simulink library "roller485lib"  (R2023a)
settings: Solver=VariableStepAuto  StartTime=0.0  StopTime=10.0  RelTol=1e-3
libraries: arduinolib x173, simulink x66
(part 3 of 6)

== system roller485lib/Basic I2C Write (using MATLAB Function)/basic angular velocity command [rpm] (using MATLAB Function) ==
  command [rpm] : Inport
  I2C Write (0x40) : arduinolib/I2C Write  I2CModule=0  Mode=Master  SlaveAddress=I2CAddress  SlaveByteOrder=BigEndian  Direction=Transmitter  RegisterAddressMode=on  RegisterAddress=0x40  SlaveDataType=uint8  DataLength=1  NoAck=off  RepeatedStart=off  OutputStatus=off  blockPlatform=ARDUINO
  MATLAB Function : MATLAB Function  TreatAsAtomicUnit=on
  x 100 : Gain  Gain=100
  wires:
  x 100/1 -> MATLAB Function/1(double_data)
  command [rpm]/1 -> x 100/1
  MATLAB Function/1(bytes) -> I2C Write (0x40)/1

== system roller485lib/Basic I2C Write (using MATLAB Function)/basic current command [A] (using MATLAB Function) ==
  command [A] : Inport
  A to mA : Gain  Gain=1000
  I2C Write (0xB0) : arduinolib/I2C Write  I2CModule=0  Mode=Master  SlaveAddress=I2CAddress  SlaveByteOrder=BigEndian  Direction=Transmitter  RegisterAddressMode=on  RegisterAddress=0xB0  SlaveDataType=uint8  DataLength=1  NoAck=off  RepeatedStart=off  OutputStatus=off  blockPlatform=ARDUINO
  MATLAB Function : MATLAB Function  TreatAsAtomicUnit=on
  x 100 : Gain  Gain=100
  wires:
  x 100/1 -> MATLAB Function/1(double_data)
  command [A]/1 -> A to mA/1
  MATLAB Function/1(bytes) -> I2C Write (0xB0)/1
  A to mA/1 -> x 100/1

== system roller485lib/Basic I2C Write (using MATLAB Function)/basic current command [mA] (using MATLAB Function) ==
  command [mA] : Inport
  I2C Write (0xB0) : arduinolib/I2C Write  I2CModule=0  Mode=Master  SlaveAddress=I2CAddress  SlaveByteOrder=BigEndian  Direction=Transmitter  RegisterAddressMode=on  RegisterAddress=0xB0  SlaveDataType=uint8  DataLength=1  NoAck=off  RepeatedStart=off  OutputStatus=off  blockPlatform=ARDUINO
  MATLAB Function : MATLAB Function  TreatAsAtomicUnit=on
  x 100 : Gain  Gain=100
  wires:
  MATLAB Function/1(bytes) -> I2C Write (0xB0)/1
  command [mA]/1 -> x 100/1
  x 100/1 -> MATLAB Function/1(double_data)

== system roller485lib/Basic I2C Write (using MATLAB Function)/basic relative angle command [deg] (using MATLAB Function) ==
  command [deg] : Inport
  Clock : Clock
  Compare To Constant : simulink/Logic and Bit Operations/Compare To Constant  relop===  const=0  OutDataTypeStr=boolean
  Enabled Subsystem (initialization angle) : Subsystem  TreatAsAtomicUnit=on
  I2C Write (0x80) : arduinolib/I2C Write  I2CModule=0  Mode=Master  SlaveAddress=I2CAddress  SlaveByteOrder=BigEndian  Direction=Transmitter  RegisterAddressMode=on  RegisterAddress=0x80  SlaveDataType=uint8  DataLength=1  NoAck=off  RepeatedStart=off  OutputStatus=off  blockPlatform=ARDUINO
  MATLAB Function : MATLAB Function  TreatAsAtomicUnit=on
  Sum : Sum  Inputs=++|
  x 100 : Gain  Gain=100
  wires:
  x 100/1 -> MATLAB Function/1(double_data)
  MATLAB Function/1(bytes) -> I2C Write (0x80)/1
  Compare To Constant/1 -> Enabled Subsystem (initialization angle)/Enable
  Clock/1 -> Compare To Constant/1
  command [deg]/1 -> Sum/2
  Enabled Subsystem (initialization angle)/1(initial angle) -> Sum/1
  Sum/1 -> x 100/1

== system roller485lib/Basic I2C Write (using MATLAB Function)/basic relative angle command [rad] (using MATLAB Function) ==
  command [rad] : Inport
  Clock : Clock
  Compare To Constant : simulink/Logic and Bit Operations/Compare To Constant  relop===  const=0  OutDataTypeStr=boolean
  Enabled Subsystem (initialization angle) : Subsystem  TreatAsAtomicUnit=on
  I2C Write (0x80) : arduinolib/I2C Write  I2CModule=0  Mode=Master  SlaveAddress=I2CAddress  SlaveByteOrder=BigEndian  Direction=Transmitter  RegisterAddressMode=on  RegisterAddress=0x80  SlaveDataType=uint8  DataLength=1  NoAck=off  RepeatedStart=off  OutputStatus=off  blockPlatform=ARDUINO
  MATLAB Function : MATLAB Function  TreatAsAtomicUnit=on
  Sum : Sum  Inputs=++|
  rad to deg : Gain  Gain=180/pi
  x 100 : Gain  Gain=100
  wires:
  Enabled Subsystem (initialization angle)/1(initial angle) -> Sum/1
  command [rad]/1 -> rad to deg/1
  Clock/1 -> Compare To Constant/1
  Compare To Constant/1 -> Enabled Subsystem (initialization angle)/Enable
  MATLAB Function/1(bytes) -> I2C Write (0x80)/1
  x 100/1 -> MATLAB Function/1(double_data)
  Sum/1 -> x 100/1
  rad to deg/1 -> Sum/2

== system roller485lib/Basic I2C Write (using MATLAB Function)/position PID (using MATLAB Function) ==
  " x 10^5 " : Gain  Gain=1e5
  D : Constant  Value=position_D
  I : Constant  Value=position_I
  I2C Write (0xA0) : arduinolib/I2C Write  I2CModule=0  Mode=Master  SlaveAddress=I2CAddress  SlaveByteOrder=BigEndian  Direction=Transmitter  RegisterAddressMode=on  RegisterAddress=0xA0  SlaveDataType=uint8  DataLength=1  NoAck=off  RepeatedStart=off  OutputStatus=off  blockPlatform=ARDUINO
  I2C Write (0xA4) : arduinolib/I2C Write  I2CModule=0  Mode=Master  SlaveAddress=I2CAddress  SlaveByteOrder=BigEndian  Direction=Transmitter  RegisterAddressMode=on  RegisterAddress=0xA4  SlaveDataType=uint8  DataLength=1  NoAck=off  RepeatedStart=off  OutputStatus=off  blockPlatform=ARDUINO
  I2C Write (0xA8) : arduinolib/I2C Write  I2CModule=0  Mode=Master  SlaveAddress=I2CAddress  SlaveByteOrder=BigEndian  Direction=Transmitter  RegisterAddressMode=on  RegisterAddress=0xA8  SlaveDataType=uint8  DataLength=1  NoAck=off  RepeatedStart=off  OutputStatus=off  blockPlatform=ARDUINO
  MATLAB Function (D) : MATLAB Function  TreatAsAtomicUnit=on
  MATLAB Function (I) : MATLAB Function  TreatAsAtomicUnit=on
  MATLAB Function (P) : MATLAB Function  TreatAsAtomicUnit=on
  P : Constant  Value=position_P
  x 10^5 : Gain  Gain=1e5
  x 10^7 : Gain  Gain=1e7
  wires:
  x 10^5/1 -> MATLAB Function (P)/1(double_data)
  MATLAB Function (P)/1(bytes) -> I2C Write (0xA0)/1
  P/1 -> x 10^5/1
  I/1 -> x 10^7/1
  MATLAB Function (I)/1(bytes) -> I2C Write (0xA4)/1
  x 10^7/1 -> MATLAB Function (I)/1(double_data)
  " x 10^5 "/1 -> MATLAB Function (D)/1(double_data)
  MATLAB Function (D)/1(bytes) -> I2C Write (0xA8)/1
  D/1 -> " x 10^5 "/1

== system roller485lib/Basic I2C Write (using MATLAB Function)/position PID (within set time) (using MATLAB Function) ==
  Clock : Clock
  Compare To Constant : simulink/Logic and Bit Operations/Compare To Constant  relop=<=  const=set_time  OutDataTypeStr=boolean
  D : Constant  Value=position_D
  Enabled Subsystem : Subsystem  TreatAsAtomicUnit=on
  I : Constant  Value=position_I
  P : Constant  Value=position_P
  wires:
  D/1 -> Enabled Subsystem/3(D)
  I/1 -> Enabled Subsystem/2(I)
  P/1 -> Enabled Subsystem/1(P)
  Compare To Constant/1 -> Enabled Subsystem/Enable
  Clock/1 -> Compare To Constant/1

== system roller485lib/Basic I2C Write (using MATLAB Function)/speed PID (using MATLAB Function) ==
  " x 10^5 " : Gain  Gain=1e5
  D : Constant  Value=speed_D
  I : Constant  Value=speed_I
  I2C Write (0x70) : arduinolib/I2C Write  I2CModule=0  Mode=Master  SlaveAddress=I2CAddress  SlaveByteOrder=BigEndian  Direction=Transmitter  RegisterAddressMode=on  RegisterAddress=0x70  SlaveDataType=uint8  DataLength=1  NoAck=off  RepeatedStart=off  OutputStatus=off  blockPlatform=ARDUINO
  I2C Write (0x74) : arduinolib/I2C Write  I2CModule=0  Mode=Master  SlaveAddress=I2CAddress  SlaveByteOrder=BigEndian  Direction=Transmitter  RegisterAddressMode=on  RegisterAddress=0x74  SlaveDataType=uint8  DataLength=1  NoAck=off  RepeatedStart=off  OutputStatus=off  blockPlatform=ARDUINO
  I2C Write (0x78) : arduinolib/I2C Write  I2CModule=0  Mode=Master  SlaveAddress=I2CAddress  SlaveByteOrder=BigEndian  Direction=Transmitter  RegisterAddressMode=on  RegisterAddress=0x78  SlaveDataType=uint8  DataLength=1  NoAck=off  RepeatedStart=off  OutputStatus=off  blockPlatform=ARDUINO
  MATLAB Function (D) : MATLAB Function  TreatAsAtomicUnit=on
  MATLAB Function (I) : MATLAB Function  TreatAsAtomicUnit=on
  MATLAB Function (P) : MATLAB Function  TreatAsAtomicUnit=on
  P : Constant  Value=speed_P
  x 10^5 : Gain  Gain=1e5
  x 10^7 : Gain  Gain=1e7
  wires:
  D/1 -> " x 10^5 "/1
  MATLAB Function (D)/1(bytes) -> I2C Write (0x78)/1
  " x 10^5 "/1 -> MATLAB Function (D)/1(double_data)
  x 10^7/1 -> MATLAB Function (I)/1(double_data)
  MATLAB Function (I)/1(bytes) -> I2C Write (0x74)/1
  I/1 -> x 10^7/1
  P/1 -> x 10^5/1
  MATLAB Function (P)/1(bytes) -> I2C Write (0x70)/1
  x 10^5/1 -> MATLAB Function (P)/1(double_data)

== system roller485lib/Basic I2C Write (using MATLAB Function)/speed PID (within set time) (using MATLAB Function) ==
  Clock : Clock
  Compare To Constant : simulink/Logic and Bit Operations/Compare To Constant  relop=<=  const=set_time  OutDataTypeStr=boolean
  D : Constant  Value=speed_D
  Enabled Subsystem : Subsystem  TreatAsAtomicUnit=on
  I : Constant  Value=speed_I
  P : Constant  Value=speed_P
  wires:
  Compare To Constant/1 -> Enabled Subsystem/Enable
  P/1 -> Enabled Subsystem/1(P)
  I/1 -> Enabled Subsystem/2(I)
  D/1 -> Enabled Subsystem/3(D)
  Clock/1 -> Compare To Constant/1

== system roller485lib/I2C Read/absolute angle detection [deg] ==
  Data Type Conversion : DataTypeConversion  OutDataTypeStr=double  SaturateOnIntegerOverflow=off  RndMeth=Floor
  I2C Read (0x90) : arduinolib/I2C Read  I2CModule=0  Mode=Master  SlaveAddress=I2CAddress  SlaveByteOrder=LittleEndian  Direction=Receiver  RegisterAddressMode=on  RegisterAddress=0x90  SlaveDataType=int32  DataLength=1  NoAck=off  RepeatedStart=off  OutputStatus=off  blockPlatform=ARDUINO  SampleTime=sample_time
  Reshape : Reshape
  x (1/100) : Gain  Gain=1/100
  deg : Outport
  wires:
  x (1/100)/1 -> Reshape/1
  I2C Read (0x90)/1 -> Data Type Conversion/1
  Data Type Conversion/1 -> x (1/100)/1
  Reshape/1 -> deg/1

== system roller485lib/I2C Read/absolute angle detection [rad] ==
  Data Type Conversion : DataTypeConversion  OutDataTypeStr=double  SaturateOnIntegerOverflow=off  RndMeth=Floor
  I2C Read (0x90) : arduinolib/I2C Read  I2CModule=0  Mode=Master  SlaveAddress=I2CAddress  SlaveByteOrder=LittleEndian  Direction=Receiver  RegisterAddressMode=on  RegisterAddress=0x90  SlaveDataType=int32  DataLength=1  NoAck=off  RepeatedStart=off  OutputStatus=off  blockPlatform=ARDUINO  SampleTime=sample_time
  Reshape : Reshape
  deg to rad : Gain  Gain=pi/180
  x (1/100) : Gain  Gain=1/100
  rad : Outport
  wires:
  x (1/100)/1 -> deg to rad/1
  deg to rad/1 -> Reshape/1
  Data Type Conversion/1 -> x (1/100)/1
  I2C Read (0x90)/1 -> Data Type Conversion/1
  Reshape/1 -> rad/1

== system roller485lib/I2C Read/angular velocity detection using LPF [rad//s] ==
  Data Type Conversion : DataTypeConversion  OutDataTypeStr=double  SaturateOnIntegerOverflow=off  RndMeth=Floor
  I2C Read (0x60) : arduinolib/I2C Read  I2CModule=0  Mode=Master  SlaveAddress=I2CAddress  SlaveByteOrder=LittleEndian  Direction=Receiver  RegisterAddressMode=on  RegisterAddress=0x60  SlaveDataType=int32  DataLength=1  NoAck=off  RepeatedStart=off  OutputStatus=off  blockPlatform=ARDUINO  SampleTime=sample_time
  Reshape : Reshape
  rpm to rad/s : Gain  Gain=2*pi/60
  x (1/100) : Gain  Gain=1/100
  rad/s : Outport
  wires:
  x (1/100)/1 -> rpm to rad/s/1
  rpm to rad/s/1 -> Reshape/1
  I2C Read (0x60)/1 -> Data Type Conversion/1
  Data Type Conversion/1 -> x (1/100)/1
  Reshape/1 -> rad/s/1

== system roller485lib/I2C Read/angular velocity detection using LPF [rpm] ==
  Data Type Conversion : DataTypeConversion  OutDataTypeStr=double  SaturateOnIntegerOverflow=off  RndMeth=Floor
  I2C Read (0x60) : arduinolib/I2C Read  I2CModule=0  Mode=Master  SlaveAddress=I2CAddress  SlaveByteOrder=LittleEndian  Direction=Receiver  RegisterAddressMode=on  RegisterAddress=0x60  SlaveDataType=int32  DataLength=1  NoAck=off  RepeatedStart=off  OutputStatus=off  blockPlatform=ARDUINO  SampleTime=sample_time
  Reshape : Reshape
  x (1/100) : Gain  Gain=1/100
  rpm : Outport
  wires:
  x (1/100)/1 -> Reshape/1
  Data Type Conversion/1 -> x (1/100)/1
  I2C Read (0x60)/1 -> Data Type Conversion/1
  Reshape/1 -> rpm/1

== system roller485lib/I2C Read/current detection [A] ==
  Data Type Conversion : DataTypeConversion  OutDataTypeStr=double  SaturateOnIntegerOverflow=off  RndMeth=Floor
  I2C Read (0xC0) : arduinolib/I2C Read  I2CModule=0  Mode=Master  SlaveAddress=I2CAddress  SlaveByteOrder=LittleEndian  Direction=Receiver  RegisterAddressMode=on  RegisterAddress=0xC0  SlaveDataType=int32  DataLength=1  NoAck=off  RepeatedStart=off  OutputStatus=off  blockPlatform=ARDUINO  SampleTime=sample_time
  Reshape : Reshape
  mA to A : Gain  Gain=1/1000
  x (1/100) : Gain  Gain=1/100
  A : Outport
  wires:
  x (1/100)/1 -> mA to A/1
  Data Type Conversion/1 -> x (1/100)/1
  mA to A/1 -> Reshape/1
  I2C Read (0xC0)/1 -> Data Type Conversion/1
  Reshape/1 -> A/1

== system roller485lib/I2C Read/current detection [mA] ==
  Data Type Conversion : DataTypeConversion  OutDataTypeStr=double  SaturateOnIntegerOverflow=off  RndMeth=Floor
  I2C Read (0xC0) : arduinolib/I2C Read  I2CModule=0  Mode=Master  SlaveAddress=I2CAddress  SlaveByteOrder=LittleEndian  Direction=Receiver  RegisterAddressMode=on  RegisterAddress=0xC0  SlaveDataType=int32  DataLength=1  NoAck=off  RepeatedStart=off  OutputStatus=off  blockPlatform=ARDUINO  SampleTime=sample_time
  Reshape : Reshape
  x (1/100) : Gain  Gain=1/100
  mA : Outport
  wires:
  Data Type Conversion/1 -> x (1/100)/1
  x (1/100)/1 -> Reshape/1
  I2C Read (0xC0)/1 -> Data Type Conversion/1
  Reshape/1 -> mA/1

== system roller485lib/I2C Read/relative angle detection [deg] ==
  Clock : Clock
  Compare To Constant : simulink/Logic and Bit Operations/Compare To Constant  relop=<=  const=set_time  OutDataTypeStr=boolean
  Data Type Conversion : DataTypeConversion  OutDataTypeStr=double  SaturateOnIntegerOverflow=off  RndMeth=Floor
  Enabled Subsystem (initialization of angle) : Subsystem  TreatAsAtomicUnit=on
  I2C Read (0x90) : arduinolib/I2C Read  I2CModule=0  Mode=Master  SlaveAddress=I2CAddress  SlaveByteOrder=LittleEndian  Direction=Receiver  RegisterAddressMode=on  RegisterAddress=0x90  SlaveDataType=int32  DataLength=1  NoAck=off  RepeatedStart=off  OutputStatus=off  blockPlatform=ARDUINO  SampleTime=sample_time
  Reshape : Reshape
  Sum : Sum  Inputs=-+|
  x (1/100) : Gain  Gain=1/100
  deg : Outport
  wires:
  Sum/1 -> x (1/100)/1
  Enabled Subsystem (initialization of angle)/1(phim(0)) -> Sum/1
  Data Type Conversion/1 -> Sum/2, Enabled Subsystem (initialization of angle)/1(phim)
  Clock/1 -> Compare To Constant/1
  x (1/100)/1 -> Reshape/1
  I2C Read (0x90)/1 -> Data Type Conversion/1
  Reshape/1 -> deg/1
  Compare To Constant/1 -> Enabled Subsystem (initialization of angle)/Enable

== system roller485lib/I2C Read/relative angle detection [rad] ==
  Clock : Clock
  Compare To Constant : simulink/Logic and Bit Operations/Compare To Constant  relop=<=  const=set_time  OutDataTypeStr=boolean
  Data Type Conversion : DataTypeConversion  OutDataTypeStr=double  SaturateOnIntegerOverflow=off  RndMeth=Floor
  Enabled Subsystem (initialization of angle) : Subsystem  TreatAsAtomicUnit=on
  I2C Read (0x90) : arduinolib/I2C Read  I2CModule=0  Mode=Master  SlaveAddress=I2CAddress  SlaveByteOrder=LittleEndian  Direction=Receiver  RegisterAddressMode=on  RegisterAddress=0x90  SlaveDataType=int32  DataLength=1  NoAck=off  RepeatedStart=off  OutputStatus=off  blockPlatform=ARDUINO  SampleTime=sample_time
  Reshape : Reshape
  Sum : Sum  Inputs=-+|
  deg to rad : Gain  Gain=pi/180
  x (1/100) : Gain  Gain=1/100
  rad : Outport
  wires:
  x (1/100)/1 -> deg to rad/1
  Clock/1 -> Compare To Constant/1
  Data Type Conversion/1 -> Enabled Subsystem (initialization of angle)/1(phim), Sum/2
  Enabled Subsystem (initialization of angle)/1(phim(0)) -> Sum/1
  Sum/1 -> x (1/100)/1
  deg to rad/1 -> Reshape/1
  I2C Read (0x90)/1 -> Data Type Conversion/1
  Reshape/1 -> rad/1
  Compare To Constant/1 -> Enabled Subsystem (initialization of angle)/Enable

== system roller485lib/I2C Read (using MATLAB Function)/absolute angle detection [deg] (using MATLAB Function) ==
  I2C Read (0x90) : arduinolib/I2C Read  I2CModule=0  Mode=Master  SlaveAddress=I2CAddress  SlaveByteOrder=BigEndian  Direction=Receiver  RegisterAddressMode=on  RegisterAddress=0x90  SlaveDataType=uint8  DataLength=4  NoAck=off  RepeatedStart=off  OutputStatus=off  blockPlatform=ARDUINO  SampleTime=sample_time
  MATLAB Function : MATLAB Function  TreatAsAtomicUnit=on
  x (1/100) : Gain  Gain=1/100
  deg : Outport
  wires:
  x (1/100)/1 -> deg/1
  MATLAB Function/1(double_data) -> x (1/100)/1
  I2C Read (0x90)/1 -> MATLAB Function/1(bytes)

== system roller485lib/I2C Read (using MATLAB Function)/absolute angle detection [rad] (using MATLAB Function) ==
  I2C Read (0x90) : arduinolib/I2C Read  I2CModule=0  Mode=Master  SlaveAddress=I2CAddress  SlaveByteOrder=BigEndian  Direction=Receiver  RegisterAddressMode=on  RegisterAddress=0x90  SlaveDataType=uint8  DataLength=4  NoAck=off  RepeatedStart=off  OutputStatus=off  blockPlatform=ARDUINO  SampleTime=sample_time
  MATLAB Function : MATLAB Function  TreatAsAtomicUnit=on
  deg to rad : Gain  Gain=pi/180
  x (1/100) : Gain  Gain=1/100
  rad : Outport
  wires:
  I2C Read (0x90)/1 -> MATLAB Function/1(bytes)
  MATLAB Function/1(double_data) -> x (1/100)/1
  x (1/100)/1 -> deg to rad/1
  deg to rad/1 -> rad/1

== system roller485lib/I2C Read (using MATLAB Function)/angular velocity detection using LPF [rad//s] (using MATLAB Function) ==
  I2C Read (0x60) : arduinolib/I2C Read  I2CModule=0  Mode=Master  SlaveAddress=I2CAddress  SlaveByteOrder=BigEndian  Direction=Receiver  RegisterAddressMode=on  RegisterAddress=0x60  SlaveDataType=uint8  DataLength=4  NoAck=off  RepeatedStart=off  OutputStatus=off  blockPlatform=ARDUINO  SampleTime=sample_time
  MATLAB Function2 : MATLAB Function  TreatAsAtomicUnit=on
  rpm to rad/s : Gain  Gain=2*pi/60
  x (1/100) : Gain  Gain=1/100
  rad/s : Outport
  wires:
  I2C Read (0x60)/1 -> MATLAB Function2/1(bytes)
  MATLAB Function2/1(double_data) -> x (1/100)/1
  x (1/100)/1 -> rpm to rad/s/1
  rpm to rad/s/1 -> rad/s/1

== system roller485lib/I2C Read (using MATLAB Function)/angular velocity detection using LPF [rpm] (using MATLAB Function) ==
  I2C Read (0x60) : arduinolib/I2C Read  I2CModule=0  Mode=Master  SlaveAddress=I2CAddress  SlaveByteOrder=BigEndian  Direction=Receiver  RegisterAddressMode=on  RegisterAddress=0x60  SlaveDataType=uint8  DataLength=4  NoAck=off  RepeatedStart=off  OutputStatus=off  blockPlatform=ARDUINO  SampleTime=sample_time
  MATLAB Function2 : MATLAB Function  TreatAsAtomicUnit=on
  x (1/100) : Gain  Gain=1/100
  rpm : Outport
  wires:
  x (1/100)/1 -> rpm/1
  MATLAB Function2/1(double_data) -> x (1/100)/1
  I2C Read (0x60)/1 -> MATLAB Function2/1(bytes)

== system roller485lib/I2C Read (using MATLAB Function)/current detection [A] (using MATLAB Function) ==
  I2C Read (0xC0) : arduinolib/I2C Read  I2CModule=0  Mode=Master  SlaveAddress=I2CAddress  SlaveByteOrder=BigEndian  Direction=Receiver  RegisterAddressMode=on  RegisterAddress=0xC0  SlaveDataType=uint8  DataLength=4  NoAck=off  RepeatedStart=off  OutputStatus=off  blockPlatform=ARDUINO  SampleTime=sample_time
  MATLAB Function : MATLAB Function  TreatAsAtomicUnit=on
  mA to A : Gain  Gain=1/1000
  x (1/100) : Gain  Gain=1/100
  A : Outport
  wires:
  x (1/100)/1 -> mA to A/1
  MATLAB Function/1(double_data) -> x (1/100)/1
  I2C Read (0xC0)/1 -> MATLAB Function/1(bytes)
  mA to A/1 -> A/1

== system roller485lib/I2C Read (using MATLAB Function)/current detection [mA] (using MATLAB Function) ==
  I2C Read (0xC0) : arduinolib/I2C Read  I2CModule=0  Mode=Master  SlaveAddress=I2CAddress  SlaveByteOrder=BigEndian  Direction=Receiver  RegisterAddressMode=on  RegisterAddress=0xC0  SlaveDataType=uint8  DataLength=4  NoAck=off  RepeatedStart=off  OutputStatus=off  blockPlatform=ARDUINO  SampleTime=sample_time
  MATLAB Function : MATLAB Function  TreatAsAtomicUnit=on
  x (1/100) : Gain  Gain=1/100
  mA : Outport
  wires:
  I2C Read (0xC0)/1 -> MATLAB Function/1(bytes)
  MATLAB Function/1(double_data) -> x (1/100)/1
  x (1/100)/1 -> mA/1

== system roller485lib/I2C Read (using MATLAB Function)/relative angle detection [deg] (using MATLAB Function) ==
  Clock : Clock
  Compare To Constant : simulink/Logic and Bit Operations/Compare To Constant  relop=<=  const=set_time  OutDataTypeStr=boolean
  Enabled Subsystem (initialization of angle) : Subsystem  TreatAsAtomicUnit=on
  I2C Read (0x90) : arduinolib/I2C Read  I2CModule=0  Mode=Master  SlaveAddress=I2CAddress  SlaveByteOrder=BigEndian  Direction=Receiver  RegisterAddressMode=on  RegisterAddress=0x90  SlaveDataType=uint8  DataLength=4  NoAck=off  RepeatedStart=off  OutputStatus=off  blockPlatform=ARDUINO  SampleTime=sample_time
  MATLAB Function : MATLAB Function  TreatAsAtomicUnit=on
  Sum : Sum  Inputs=-+|
  x (1/100) : Gain  Gain=1/100
  deg : Outport
  wires:
  Sum/1 -> x (1/100)/1
  Enabled Subsystem (initialization of angle)/1(phim(0)) -> Sum/1
  MATLAB Function/1(double_data) -> Sum/2, Enabled Subsystem (initialization of angle)/1(phim)
  Compare To Constant/1 -> Enabled Subsystem (initialization of angle)/Enable
  I2C Read (0x90)/1 -> MATLAB Function/1(bytes)
  x (1/100)/1 -> deg/1
  Clock/1 -> Compare To Constant/1

== system roller485lib/I2C Read (using MATLAB Function)/relative angle detection [rad] (using MATLAB Function) ==
  Clock : Clock
  Compare To Constant : simulink/Logic and Bit Operations/Compare To Constant  relop=<=  const=set_time  OutDataTypeStr=boolean
  Enabled Subsystem (initialization of angle) : Subsystem  TreatAsAtomicUnit=on
  I2C Read (0x90) : arduinolib/I2C Read  I2CModule=0  Mode=Master  SlaveAddress=I2CAddress  SlaveByteOrder=BigEndian  Direction=Receiver  RegisterAddressMode=on  RegisterAddress=0x90  SlaveDataType=uint8  DataLength=4  NoAck=off  RepeatedStart=off  OutputStatus=off  blockPlatform=ARDUINO  SampleTime=sample_time
  MATLAB Function : MATLAB Function  TreatAsAtomicUnit=on
  Sum : Sum  Inputs=-+|
  deg to rad : Gain  Gain=pi/180
  x (1/100) : Gain  Gain=1/100
  deg : Outport
  wires:
  x (1/100)/1 -> deg to rad/1
  I2C Read (0x90)/1 -> MATLAB Function/1(bytes)
  Compare To Constant/1 -> Enabled Subsystem (initialization of angle)/Enable
  MATLAB Function/1(double_data) -> Enabled Subsystem (initialization of angle)/1(phim), Sum/2
  Enabled Subsystem (initialization of angle)/1(phim(0)) -> Sum/1
  Sum/1 -> x (1/100)/1
  deg to rad/1 -> deg/1
  Clock/1 -> Compare To Constant/1

== system roller485lib/I2C Write/absolute angle command [deg] ==
  command [deg] : Inport
  Clock1 : Clock
  Clock2 : Clock
  Compare To Constant1 : simulink/Logic and Bit Operations/Compare To Constant  relop=<=  const=set_time1  OutDataTypeStr=boolean
  Compare To Constant2 : simulink/Logic and Bit Operations/Compare To Constant  relop=<=  const=set_time2  OutDataTypeStr=boolean
  D : Constant  Value=position_D
  Data Type Conversion : DataTypeConversion  OutDataTypeStr=uint32  SaturateOnIntegerOverflow=off  RndMeth=Floor
  Enabled Subsystem (PID setting) : Subsystem  TreatAsAtomicUnit=on
  Enabled Subsystem (mode setting) : Subsystem  TreatAsAtomicUnit=on
  I : Constant  Value=position_I
  I2C Write (0x80) : arduinolib/I2C Write  I2CModule=0  Mode=Master  SlaveAddress=I2CAddress  SlaveByteOrder=LittleEndian  Direction=Transmitter  RegisterAddressMode=on  RegisterAddress=0x80  SlaveDataType=uint8  DataLength=1  NoAck=off  RepeatedStart=off  OutputStatus=off  blockPlatform=ARDUINO
  P : Constant  Value=position_P
  position mode : Constant  Value=2
  x 100 : Gain  Gain=100
  wires:
  P/1 -> Enabled Subsystem (PID setting)/1(P)
  Clock1/1 -> Compare To Constant1/1
  position mode/1 -> Enabled Subsystem (mode setting)/1(mode)
  I/1 -> Enabled Subsystem (PID setting)/2(I)
  x 100/1 -> Data Type Conversion/1
  D/1 -> Enabled Subsystem (PID setting)/3(D)
  Compare To Constant2/1 -> Enabled Subsystem (PID setting)/Enable
  Compare To Constant1/1 -> Enabled Subsystem (mode setting)/Enable
  Clock2/1 -> Compare To Constant2/1
  Data Type Conversion/1 -> I2C Write (0x80)/1
  command [deg]/1 -> x 100/1

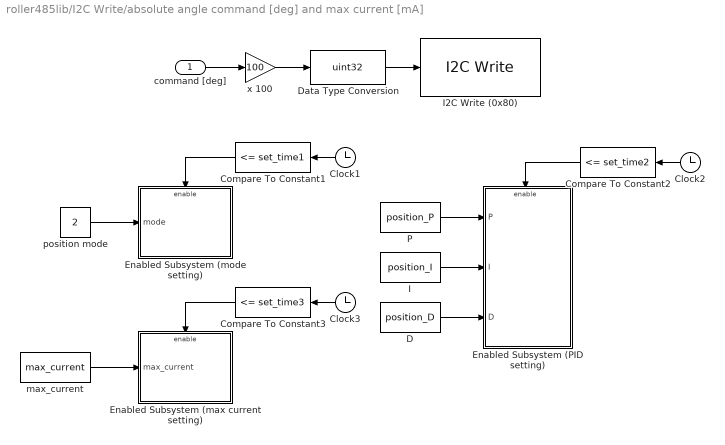
== system roller485lib/I2C Write/absolute angle command [deg] and max current [mA] ==
  command [deg] : Inport
  Clock1 : Clock
  Clock2 : Clock
  Clock3 : Clock
  Compare To Constant1 : simulink/Logic and Bit Operations/Compare To Constant  relop=<=  const=set_time1  OutDataTypeStr=boolean
  Compare To Constant2 : simulink/Logic and Bit Operations/Compare To Constant  relop=<=  const=set_time2  OutDataTypeStr=boolean
  Compare To Constant3 : simulink/Logic and Bit Operations/Compare To Constant  relop=<=  const=set_time3  OutDataTypeStr=boolean
  D : Constant  Value=position_D
  Data Type Conversion : DataTypeConversion  OutDataTypeStr=uint32  SaturateOnIntegerOverflow=off  RndMeth=Floor
  Enabled Subsystem (PID setting) : Subsystem  TreatAsAtomicUnit=on
  Enabled Subsystem (max current setting) : Subsystem  TreatAsAtomicUnit=on
  Enabled Subsystem (mode setting) : Subsystem  TreatAsAtomicUnit=on
  I : Constant  Value=position_I
  I2C Write (0x80) : arduinolib/I2C Write  I2CModule=0  Mode=Master  SlaveAddress=I2CAddress  SlaveByteOrder=LittleEndian  Direction=Transmitter  RegisterAddressMode=on  RegisterAddress=0x80  SlaveDataType=uint8  DataLength=1  NoAck=off  RepeatedStart=off  OutputStatus=off  blockPlatform=ARDUINO
  P : Constant  Value=position_P
  max_current : Constant  Value=max_current
  position mode : Constant  Value=2
  x 100 : Gain  Gain=100
  wires:
  P/1 -> Enabled Subsystem (PID setting)/1(P)
  Clock1/1 -> Compare To Constant1/1
  position mode/1 -> Enabled Subsystem (mode setting)/1(mode)
  I/1 -> Enabled Subsystem (PID setting)/2(I)
  Clock3/1 -> Compare To Constant3/1
  x 100/1 -> Data Type Conversion/1
  Compare To Constant3/1 -> Enabled Subsystem (max current setting)/Enable
  D/1 -> Enabled Subsystem (PID setting)/3(D)
  Compare To Constant2/1 -> Enabled Subsystem (PID setting)/Enable
  Compare To Constant1/1 -> Enabled Subsystem (mode setting)/Enable
  Clock2/1 -> Compare To Constant2/1
  max_current/1 -> Enabled Subsystem (max current setting)/1(max_current)
  Data Type Conversion/1 -> I2C Write (0x80)/1
  command [deg]/1 -> x 100/1

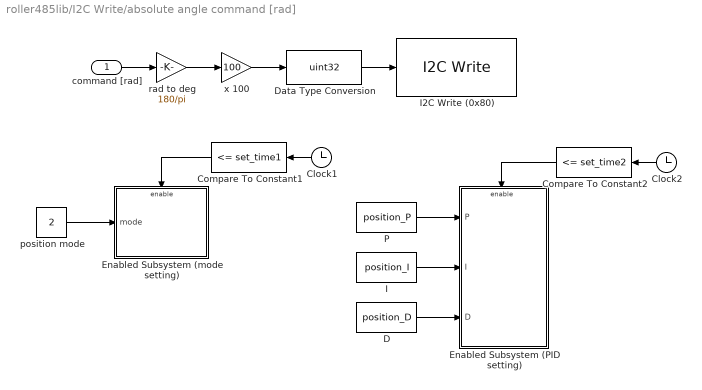
== system roller485lib/I2C Write/absolute angle command [rad] ==
  command [rad] : Inport
  Clock1 : Clock
  Clock2 : Clock
  Compare To Constant1 : simulink/Logic and Bit Operations/Compare To Constant  relop=<=  const=set_time1  OutDataTypeStr=boolean
  Compare To Constant2 : simulink/Logic and Bit Operations/Compare To Constant  relop=<=  const=set_time2  OutDataTypeStr=boolean
  D : Constant  Value=position_D
  Data Type Conversion : DataTypeConversion  OutDataTypeStr=uint32  SaturateOnIntegerOverflow=off  RndMeth=Floor
  Enabled Subsystem (PID setting) : Subsystem  TreatAsAtomicUnit=on
  Enabled Subsystem (mode setting) : Subsystem  TreatAsAtomicUnit=on
  I : Constant  Value=position_I
  I2C Write (0x80) : arduinolib/I2C Write  I2CModule=0  Mode=Master  SlaveAddress=I2CAddress  SlaveByteOrder=LittleEndian  Direction=Transmitter  RegisterAddressMode=on  RegisterAddress=0x80  SlaveDataType=uint8  DataLength=1  NoAck=off  RepeatedStart=off  OutputStatus=off  blockPlatform=ARDUINO
  P : Constant  Value=position_P
  position mode : Constant  Value=2
  rad to deg : Gain  Gain=180/pi
  x 100 : Gain  Gain=100
  wires:
  P/1 -> Enabled Subsystem (PID setting)/1(P)
  Clock1/1 -> Compare To Constant1/1
  position mode/1 -> Enabled Subsystem (mode setting)/1(mode)
  I/1 -> Enabled Subsystem (PID setting)/2(I)
  x 100/1 -> Data Type Conversion/1
  command [rad]/1 -> rad to deg/1
  D/1 -> Enabled Subsystem (PID setting)/3(D)
  Compare To Constant2/1 -> Enabled Subsystem (PID setting)/Enable
  Compare To Constant1/1 -> Enabled Subsystem (mode setting)/Enable
  Clock2/1 -> Compare To Constant2/1
  Data Type Conversion/1 -> I2C Write (0x80)/1
  rad to deg/1 -> x 100/1

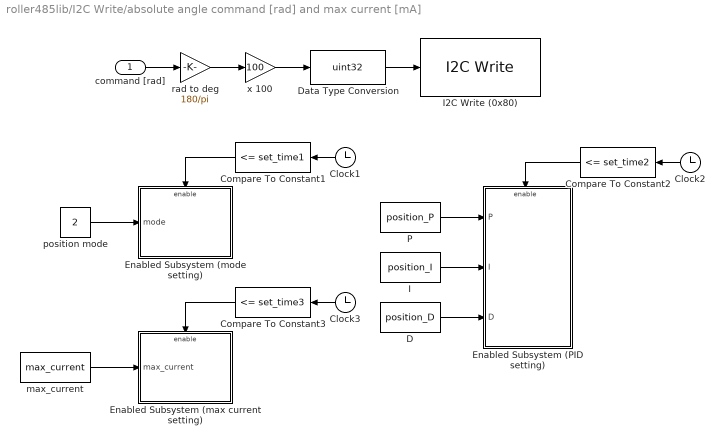
== system roller485lib/I2C Write/absolute angle command [rad] and max current [mA] ==
  command [rad] : Inport
  Clock1 : Clock
  Clock2 : Clock
  Clock3 : Clock
  Compare To Constant1 : simulink/Logic and Bit Operations/Compare To Constant  relop=<=  const=set_time1  OutDataTypeStr=boolean
  Compare To Constant2 : simulink/Logic and Bit Operations/Compare To Constant  relop=<=  const=set_time2  OutDataTypeStr=boolean
  Compare To Constant3 : simulink/Logic and Bit Operations/Compare To Constant  relop=<=  const=set_time3  OutDataTypeStr=boolean
  D : Constant  Value=position_D
  Data Type Conversion : DataTypeConversion  OutDataTypeStr=uint32  SaturateOnIntegerOverflow=off  RndMeth=Floor
  Enabled Subsystem (PID setting) : Subsystem  TreatAsAtomicUnit=on
  Enabled Subsystem (max current setting) : Subsystem  TreatAsAtomicUnit=on
  Enabled Subsystem (mode setting) : Subsystem  TreatAsAtomicUnit=on
  I : Constant  Value=position_I
  I2C Write (0x80) : arduinolib/I2C Write  I2CModule=0  Mode=Master  SlaveAddress=I2CAddress  SlaveByteOrder=LittleEndian  Direction=Transmitter  RegisterAddressMode=on  RegisterAddress=0x80  SlaveDataType=uint8  DataLength=1  NoAck=off  RepeatedStart=off  OutputStatus=off  blockPlatform=ARDUINO
  P : Constant  Value=position_P
  max_current : Constant  Value=max_current
  position mode : Constant  Value=2
  rad to deg : Gain  Gain=180/pi
  x 100 : Gain  Gain=100
  wires:
  command [rad]/1 -> rad to deg/1
  rad to deg/1 -> x 100/1
  Data Type Conversion/1 -> I2C Write (0x80)/1
  x 100/1 -> Data Type Conversion/1
  P/1 -> Enabled Subsystem (PID setting)/1(P)
  Clock1/1 -> Compare To Constant1/1
  Compare To Constant2/1 -> Enabled Subsystem (PID setting)/Enable
  I/1 -> Enabled Subsystem (PID setting)/2(I)
  D/1 -> Enabled Subsystem (PID setting)/3(D)
  Compare To Constant3/1 -> Enabled Subsystem (max current setting)/Enable
  Clock3/1 -> Compare To Constant3/1
  position mode/1 -> Enabled Subsystem (mode setting)/1(mode)
  max_current/1 -> Enabled Subsystem (max current setting)/1(max_current)
  Compare To Constant1/1 -> Enabled Subsystem (mode setting)/Enable
  Clock2/1 -> Compare To Constant2/1

== system roller485lib/I2C Write/angular velocity command [rad//s] ==
  command [rad/s] : Inport
  Clock1 : Clock
  Clock2 : Clock
  Compare To Constant1 : simulink/Logic and Bit Operations/Compare To Constant  relop=<=  const=set_time1  OutDataTypeStr=boolean
  Compare To Constant2 : simulink/Logic and Bit Operations/Compare To Constant  relop=<=  const=set_time2  OutDataTypeStr=boolean
  D : Constant  Value=speed_D
  Data Type Conversion : DataTypeConversion  OutDataTypeStr=uint32  SaturateOnIntegerOverflow=off  RndMeth=Floor
  Enabled Subsystem (PID setting) : Subsystem  TreatAsAtomicUnit=on
  Enabled Subsystem (mode setting) : Subsystem  TreatAsAtomicUnit=on
  I : Constant  Value=speed_I
  I2C Write (0x40) : arduinolib/I2C Write  I2CModule=0  Mode=Master  SlaveAddress=I2CAddress  SlaveByteOrder=LittleEndian  Direction=Transmitter  RegisterAddressMode=on  RegisterAddress=0x40  SlaveDataType=uint8  DataLength=1  NoAck=off  RepeatedStart=off  OutputStatus=off  blockPlatform=ARDUINO
  P : Constant  Value=speed_P
  rad/s to rpm : Gain  Gain=60/(2*pi)
  speed mode : Constant
  x 100 : Gain  Gain=100
  wires:
  command [rad/s]/1 -> rad/s to rpm/1
  rad/s to rpm/1 -> x 100/1
  Data Type Conversion/1 -> I2C Write (0x40)/1
  I/1 -> Enabled Subsystem (PID setting)/2(I)
  P/1 -> Enabled Subsystem (PID setting)/1(P)
  speed mode/1 -> Enabled Subsystem (mode setting)/1(mode)
  D/1 -> Enabled Subsystem (PID setting)/3(D)
  x 100/1 -> Data Type Conversion/1
  Compare To Constant1/1 -> Enabled Subsystem (mode setting)/Enable
  Clock2/1 -> Compare To Constant2/1
  Clock1/1 -> Compare To Constant1/1
  Compare To Constant2/1 -> Enabled Subsystem (PID setting)/Enable

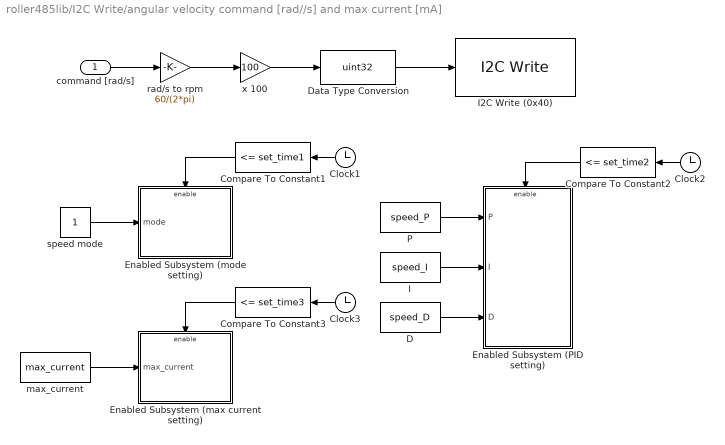
== system roller485lib/I2C Write/angular velocity command [rad//s] and max current [mA] ==
  command [rad/s] : Inport
  Clock1 : Clock
  Clock2 : Clock
  Clock3 : Clock
  Compare To Constant1 : simulink/Logic and Bit Operations/Compare To Constant  relop=<=  const=set_time1  OutDataTypeStr=boolean
  Compare To Constant2 : simulink/Logic and Bit Operations/Compare To Constant  relop=<=  const=set_time2  OutDataTypeStr=boolean
  Compare To Constant3 : simulink/Logic and Bit Operations/Compare To Constant  relop=<=  const=set_time3  OutDataTypeStr=boolean
  D : Constant  Value=speed_D
  Data Type Conversion : DataTypeConversion  OutDataTypeStr=uint32  SaturateOnIntegerOverflow=off  RndMeth=Floor
  Enabled Subsystem (PID setting) : Subsystem  TreatAsAtomicUnit=on
  Enabled Subsystem (max current setting) : Subsystem  TreatAsAtomicUnit=on
  Enabled Subsystem (mode setting) : Subsystem  TreatAsAtomicUnit=on
  I : Constant  Value=speed_I
  I2C Write (0x40) : arduinolib/I2C Write  I2CModule=0  Mode=Master  SlaveAddress=I2CAddress  SlaveByteOrder=LittleEndian  Direction=Transmitter  RegisterAddressMode=on  RegisterAddress=0x40  SlaveDataType=uint8  DataLength=1  NoAck=off  RepeatedStart=off  OutputStatus=off  blockPlatform=ARDUINO
  P : Constant  Value=speed_P
  max_current : Constant  Value=max_current
  rad/s to rpm : Gain  Gain=60/(2*pi)
  speed mode : Constant
  x 100 : Gain  Gain=100
  wires:
  command [rad/s]/1 -> rad/s to rpm/1
  rad/s to rpm/1 -> x 100/1
  Data Type Conversion/1 -> I2C Write (0x40)/1
  x 100/1 -> Data Type Conversion/1
  Clock2/1 -> Compare To Constant2/1
  Clock1/1 -> Compare To Constant1/1
  Clock3/1 -> Compare To Constant3/1
  Compare To Constant2/1 -> Enabled Subsystem (PID setting)/Enable
  D/1 -> Enabled Subsystem (PID setting)/3(D)
  I/1 -> Enabled Subsystem (PID setting)/2(I)
  P/1 -> Enabled Subsystem (PID setting)/1(P)
  max_current/1 -> Enabled Subsystem (max current setting)/1(max_current)
  speed mode/1 -> Enabled Subsystem (mode setting)/1(mode)
  Compare To Constant1/1 -> Enabled Subsystem (mode setting)/Enable
  Compare To Constant3/1 -> Enabled Subsystem (max current setting)/Enable

== system roller485lib/I2C Write/angular velocity command [rpm] ==
  command [rpm] : Inport
  Clock1 : Clock
  Clock2 : Clock
  Compare To Constant1 : simulink/Logic and Bit Operations/Compare To Constant  relop=<=  const=set_time1  OutDataTypeStr=boolean
  Compare To Constant2 : simulink/Logic and Bit Operations/Compare To Constant  relop=<=  const=set_time2  OutDataTypeStr=boolean
  D : Constant  Value=speed_D
  Data Type Conversion : DataTypeConversion  OutDataTypeStr=uint32  SaturateOnIntegerOverflow=off  RndMeth=Floor
  Enabled Subsystem (PID setting) : Subsystem  TreatAsAtomicUnit=on
  Enabled Subsystem (mode setting) : Subsystem  TreatAsAtomicUnit=on
  I : Constant  Value=speed_I
  I2C Write (0x40) : arduinolib/I2C Write  I2CModule=0  Mode=Master  SlaveAddress=I2CAddress  SlaveByteOrder=LittleEndian  Direction=Transmitter  RegisterAddressMode=on  RegisterAddress=0x40  SlaveDataType=uint8  DataLength=1  NoAck=off  RepeatedStart=off  OutputStatus=off  blockPlatform=ARDUINO
  P : Constant  Value=speed_P
  speed mode : Constant
  x 100 : Gain  Gain=100
  wires:
  Compare To Constant2/1 -> Enabled Subsystem (PID setting)/Enable
  Clock1/1 -> Compare To Constant1/1
  Clock2/1 -> Compare To Constant2/1
  Compare To Constant1/1 -> Enabled Subsystem (mode setting)/Enable
  x 100/1 -> Data Type Conversion/1
  D/1 -> Enabled Subsystem (PID setting)/3(D)
  speed mode/1 -> Enabled Subsystem (mode setting)/1(mode)
  P/1 -> Enabled Subsystem (PID setting)/1(P)
  I/1 -> Enabled Subsystem (PID setting)/2(I)
  Data Type Conversion/1 -> I2C Write (0x40)/1
  command [rpm]/1 -> x 100/1

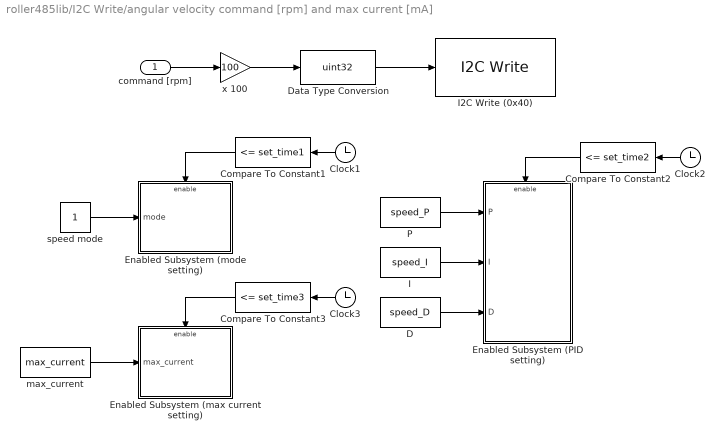
== system roller485lib/I2C Write/angular velocity command [rpm] and max current [mA] ==
  command [rpm] : Inport
  Clock1 : Clock
  Clock2 : Clock
  Clock3 : Clock
  Compare To Constant1 : simulink/Logic and Bit Operations/Compare To Constant  relop=<=  const=set_time1  OutDataTypeStr=boolean
  Compare To Constant2 : simulink/Logic and Bit Operations/Compare To Constant  relop=<=  const=set_time2  OutDataTypeStr=boolean
  Compare To Constant3 : simulink/Logic and Bit Operations/Compare To Constant  relop=<=  const=set_time3  OutDataTypeStr=boolean
  D : Constant  Value=speed_D
  Data Type Conversion : DataTypeConversion  OutDataTypeStr=uint32  SaturateOnIntegerOverflow=off  RndMeth=Floor
  Enabled Subsystem (PID setting) : Subsystem  TreatAsAtomicUnit=on
  Enabled Subsystem (max current setting) : Subsystem  TreatAsAtomicUnit=on
  Enabled Subsystem (mode setting) : Subsystem  TreatAsAtomicUnit=on
  I : Constant  Value=speed_I
  I2C Write (0x40) : arduinolib/I2C Write  I2CModule=0  Mode=Master  SlaveAddress=I2CAddress  SlaveByteOrder=LittleEndian  Direction=Transmitter  RegisterAddressMode=on  RegisterAddress=0x40  SlaveDataType=uint8  DataLength=1  NoAck=off  RepeatedStart=off  OutputStatus=off  blockPlatform=ARDUINO
  P : Constant  Value=speed_P
  max_current : Constant  Value=max_current
  speed mode : Constant
  x 100 : Gain  Gain=100
  wires:
  x 100/1 -> Data Type Conversion/1
  D/1 -> Enabled Subsystem (PID setting)/3(D)
  speed mode/1 -> Enabled Subsystem (mode setting)/1(mode)
  P/1 -> Enabled Subsystem (PID setting)/1(P)
  I/1 -> Enabled Subsystem (PID setting)/2(I)
  Data Type Conversion/1 -> I2C Write (0x40)/1
  command [rpm]/1 -> x 100/1
  max_current/1 -> Enabled Subsystem (max current setting)/1(max_current)
  Compare To Constant3/1 -> Enabled Subsystem (max current setting)/Enable
  Compare To Constant1/1 -> Enabled Subsystem (mode setting)/Enable
  Clock2/1 -> Compare To Constant2/1
  Clock1/1 -> Compare To Constant1/1
  Compare To Constant2/1 -> Enabled Subsystem (PID setting)/Enable
  Clock3/1 -> Compare To Constant3/1

== system roller485lib/I2C Write/current command [A] ==
  command [A] : Inport
  A to mA : Gain  Gain=1000
  "Clock " : Clock
  Compare To Constant : simulink/Logic and Bit Operations/Compare To Constant  relop=<=  const=set_time  OutDataTypeStr=boolean
  Data Type Conversion : DataTypeConversion  OutDataTypeStr=uint32  SaturateOnIntegerOverflow=off  RndMeth=Floor
  Enabled Subsystem (mode setting) : Subsystem  TreatAsAtomicUnit=on
  I2C Write (0xB0) : arduinolib/I2C Write  I2CModule=0  Mode=Master  SlaveAddress=I2CAddress  SlaveByteOrder=LittleEndian  Direction=Transmitter  RegisterAddressMode=on  RegisterAddress=0xB0  SlaveDataType=uint8  DataLength=1  NoAck=off  RepeatedStart=off  OutputStatus=off  blockPlatform=ARDUINO
  current mode : Constant  Value=3
  x 100 : Gain  Gain=100
  wires:
  x 100/1 -> Data Type Conversion/1
  command [A]/1 -> A to mA/1
  Data Type Conversion/1 -> I2C Write (0xB0)/1
  "Clock "/1 -> Compare To Constant/1
  Compare To Constant/1 -> Enabled Subsystem (mode setting)/Enable
  current mode/1 -> Enabled Subsystem (mode setting)/1(mode)
  A to mA/1 -> x 100/1

== system roller485lib/I2C Write/current command [mA] ==
  command [mA] : Inport
  "Clock " : Clock
  Compare To Constant : simulink/Logic and Bit Operations/Compare To Constant  relop=<=  const=set_time  OutDataTypeStr=boolean
  Data Type Conversion : DataTypeConversion  OutDataTypeStr=uint32  SaturateOnIntegerOverflow=off  RndMeth=Floor
  Enabled Subsystem (mode setting) : Subsystem  TreatAsAtomicUnit=on
  I2C Write (0xB0) : arduinolib/I2C Write  I2CModule=0  Mode=Master  SlaveAddress=I2CAddress  SlaveByteOrder=LittleEndian  Direction=Transmitter  RegisterAddressMode=on  RegisterAddress=0xB0  SlaveDataType=uint8  DataLength=1  NoAck=off  RepeatedStart=off  OutputStatus=off  blockPlatform=ARDUINO
  current mode : Constant  Value=3
  x 100 : Gain  Gain=100
  wires:
  current mode/1 -> Enabled Subsystem (mode setting)/1(mode)
  Compare To Constant/1 -> Enabled Subsystem (mode setting)/Enable
  "Clock "/1 -> Compare To Constant/1
  Data Type Conversion/1 -> I2C Write (0xB0)/1
  command [mA]/1 -> x 100/1
  x 100/1 -> Data Type Conversion/1

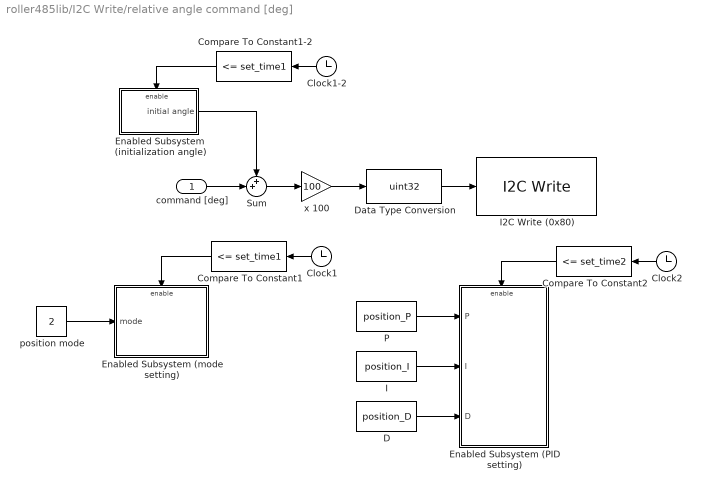
== system roller485lib/I2C Write/relative angle command [deg] ==
  command [deg] : Inport
  Clock1 : Clock
  Clock1-2 : Clock
  Clock2 : Clock
  Compare To Constant1 : simulink/Logic and Bit Operations/Compare To Constant  relop=<=  const=set_time1  OutDataTypeStr=boolean
  Compare To Constant1-2 : simulink/Logic and Bit Operations/Compare To Constant  relop=<=  const=set_time1  OutDataTypeStr=boolean
  Compare To Constant2 : simulink/Logic and Bit Operations/Compare To Constant  relop=<=  const=set_time2  OutDataTypeStr=boolean
  D : Constant  Value=position_D
  Data Type Conversion : DataTypeConversion  OutDataTypeStr=uint32  SaturateOnIntegerOverflow=off  RndMeth=Floor
  Enabled Subsystem (PID setting) : Subsystem  TreatAsAtomicUnit=on
  Enabled Subsystem (initialization angle) : Subsystem  TreatAsAtomicUnit=on
  Enabled Subsystem (mode setting) : Subsystem  TreatAsAtomicUnit=on
  I : Constant  Value=position_I
  I2C Write (0x80) : arduinolib/I2C Write  I2CModule=0  Mode=Master  SlaveAddress=I2CAddress  SlaveByteOrder=LittleEndian  Direction=Transmitter  RegisterAddressMode=on  RegisterAddress=0x80  SlaveDataType=uint8  DataLength=1  NoAck=off  RepeatedStart=off  OutputStatus=off  blockPlatform=ARDUINO
  P : Constant  Value=position_P
  Sum : Sum  Inputs=++|
  position mode : Constant  Value=2
  x 100 : Gain  Gain=100
  wires:
  Compare To Constant1-2/1 -> Enabled Subsystem (initialization angle)/Enable
  command [deg]/1 -> Sum/2
  Enabled Subsystem (initialization angle)/1(initial angle) -> Sum/1
  x 100/1 -> Data Type Conversion/1
  Sum/1 -> x 100/1
  Compare To Constant2/1 -> Enabled Subsystem (PID setting)/Enable
  position mode/1 -> Enabled Subsystem (mode setting)/1(mode)
  P/1 -> Enabled Subsystem (PID setting)/1(P)
  Clock1/1 -> Compare To Constant1/1
  Compare To Constant1/1 -> Enabled Subsystem (mode setting)/Enable
  Data Type Conversion/1 -> I2C Write (0x80)/1
  D/1 -> Enabled Subsystem (PID setting)/3(D)
  I/1 -> Enabled Subsystem (PID setting)/2(I)
  Clock2/1 -> Compare To Constant2/1
  Clock1-2/1 -> Compare To Constant1-2/1

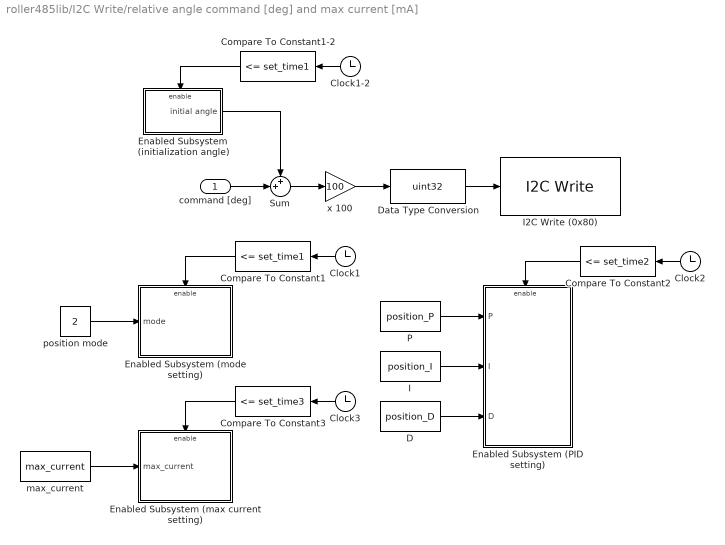
== system roller485lib/I2C Write/relative angle command [deg] and max current [mA] ==
  command [deg] : Inport
  Clock1 : Clock
  Clock1-2 : Clock
  Clock2 : Clock
  Clock3 : Clock
  Compare To Constant1 : simulink/Logic and Bit Operations/Compare To Constant  relop=<=  const=set_time1  OutDataTypeStr=boolean
  Compare To Constant1-2 : simulink/Logic and Bit Operations/Compare To Constant  relop=<=  const=set_time1  OutDataTypeStr=boolean
  Compare To Constant2 : simulink/Logic and Bit Operations/Compare To Constant  relop=<=  const=set_time2  OutDataTypeStr=boolean
  Compare To Constant3 : simulink/Logic and Bit Operations/Compare To Constant  relop=<=  const=set_time3  OutDataTypeStr=boolean
  D : Constant  Value=position_D
  Data Type Conversion : DataTypeConversion  OutDataTypeStr=uint32  SaturateOnIntegerOverflow=off  RndMeth=Floor
  Enabled Subsystem (PID setting) : Subsystem  TreatAsAtomicUnit=on
  Enabled Subsystem (initialization angle) : Subsystem  TreatAsAtomicUnit=on
  Enabled Subsystem (max current setting) : Subsystem  TreatAsAtomicUnit=on
  Enabled Subsystem (mode setting) : Subsystem  TreatAsAtomicUnit=on
  I : Constant  Value=position_I
  I2C Write (0x80) : arduinolib/I2C Write  I2CModule=0  Mode=Master  SlaveAddress=I2CAddress  SlaveByteOrder=LittleEndian  Direction=Transmitter  RegisterAddressMode=on  RegisterAddress=0x80  SlaveDataType=uint8  DataLength=1  NoAck=off  RepeatedStart=off  OutputStatus=off  blockPlatform=ARDUINO
  P : Constant  Value=position_P
  Sum : Sum  Inputs=++|
  max_current : Constant  Value=max_current
  position mode : Constant  Value=2
  x 100 : Gain  Gain=100
  wires:
  Compare To Constant1-2/1 -> Enabled Subsystem (initialization angle)/Enable
  command [deg]/1 -> Sum/2
  Enabled Subsystem (initialization angle)/1(initial angle) -> Sum/1
  x 100/1 -> Data Type Conversion/1
  Sum/1 -> x 100/1
  max_current/1 -> Enabled Subsystem (max current setting)/1(max_current)
  Compare To Constant2/1 -> Enabled Subsystem (PID setting)/Enable
  Compare To Constant3/1 -> Enabled Subsystem (max current setting)/Enable
  position mode/1 -> Enabled Subsystem (mode setting)/1(mode)
  P/1 -> Enabled Subsystem (PID setting)/1(P)
  Clock1/1 -> Compare To Constant1/1
  Compare To Constant1/1 -> Enabled Subsystem (mode setting)/Enable
  Data Type Conversion/1 -> I2C Write (0x80)/1
  D/1 -> Enabled Subsystem (PID setting)/3(D)
  I/1 -> Enabled Subsystem (PID setting)/2(I)
  Clock3/1 -> Compare To Constant3/1
  Clock2/1 -> Compare To Constant2/1
  Clock1-2/1 -> Compare To Constant1-2/1

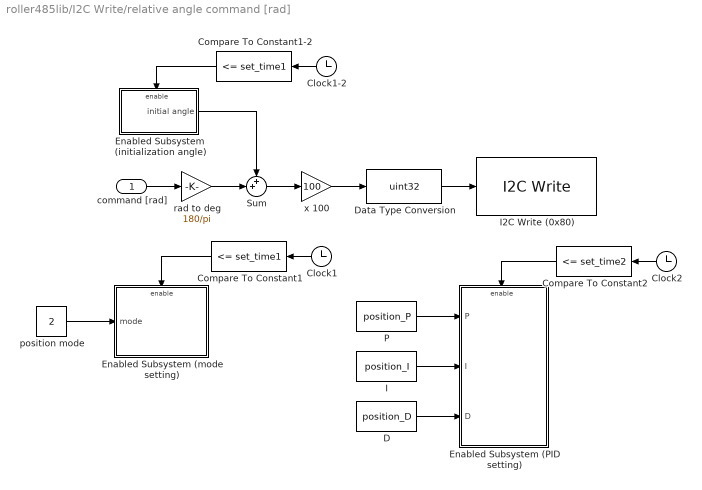
== system roller485lib/I2C Write/relative angle command [rad] ==
  command [rad] : Inport
  Clock1 : Clock
  Clock1-2 : Clock
  Clock2 : Clock
  Compare To Constant1 : simulink/Logic and Bit Operations/Compare To Constant  relop=<=  const=set_time1  OutDataTypeStr=boolean
  Compare To Constant1-2 : simulink/Logic and Bit Operations/Compare To Constant  relop=<=  const=set_time1  OutDataTypeStr=boolean
  Compare To Constant2 : simulink/Logic and Bit Operations/Compare To Constant  relop=<=  const=set_time2  OutDataTypeStr=boolean
  D : Constant  Value=position_D
  Data Type Conversion : DataTypeConversion  OutDataTypeStr=uint32  SaturateOnIntegerOverflow=off  RndMeth=Floor
  Enabled Subsystem (PID setting) : Subsystem  TreatAsAtomicUnit=on
  Enabled Subsystem (initialization angle) : Subsystem  TreatAsAtomicUnit=on
  Enabled Subsystem (mode setting) : Subsystem  TreatAsAtomicUnit=on
  I : Constant  Value=position_I
  I2C Write (0x80) : arduinolib/I2C Write  I2CModule=0  Mode=Master  SlaveAddress=I2CAddress  SlaveByteOrder=LittleEndian  Direction=Transmitter  RegisterAddressMode=on  RegisterAddress=0x80  SlaveDataType=uint8  DataLength=1  NoAck=off  RepeatedStart=off  OutputStatus=off  blockPlatform=ARDUINO
  P : Constant  Value=position_P
  Sum : Sum  Inputs=++|
  position mode : Constant  Value=2
  rad to deg : Gain  Gain=180/pi
  x 100 : Gain  Gain=100
  wires:
  Compare To Constant1-2/1 -> Enabled Subsystem (initialization angle)/Enable
  command [rad]/1 -> rad to deg/1
  rad to deg/1 -> Sum/2
  Enabled Subsystem (initialization angle)/1(initial angle) -> Sum/1
  x 100/1 -> Data Type Conversion/1
  Sum/1 -> x 100/1
  Compare To Constant2/1 -> Enabled Subsystem (PID setting)/Enable
  position mode/1 -> Enabled Subsystem (mode setting)/1(mode)
  P/1 -> Enabled Subsystem (PID setting)/1(P)
  Clock1/1 -> Compare To Constant1/1
  Compare To Constant1/1 -> Enabled Subsystem (mode setting)/Enable
  Data Type Conversion/1 -> I2C Write (0x80)/1
  D/1 -> Enabled Subsystem (PID setting)/3(D)
  I/1 -> Enabled Subsystem (PID setting)/2(I)
  Clock2/1 -> Compare To Constant2/1
  Clock1-2/1 -> Compare To Constant1-2/1

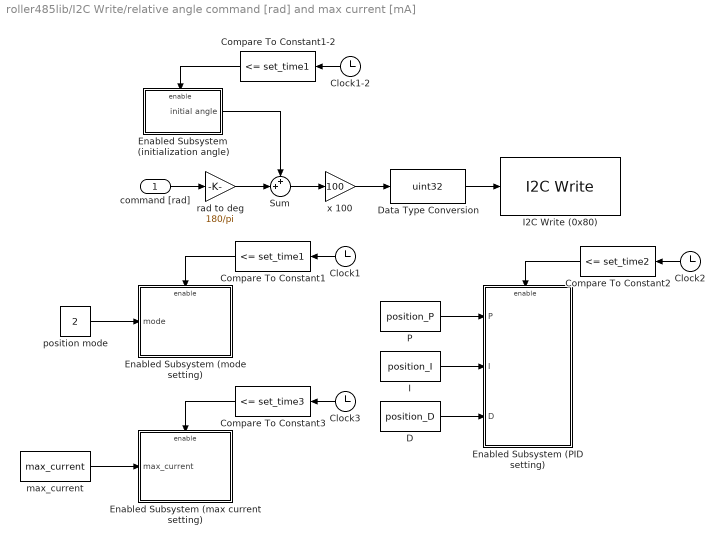
== system roller485lib/I2C Write/relative angle command [rad] and max current [mA] ==
  command [rad] : Inport
  Clock1 : Clock
  Clock1-2 : Clock
  Clock2 : Clock
  Clock3 : Clock
  Compare To Constant1 : simulink/Logic and Bit Operations/Compare To Constant  relop=<=  const=set_time1  OutDataTypeStr=boolean
  Compare To Constant1-2 : simulink/Logic and Bit Operations/Compare To Constant  relop=<=  const=set_time1  OutDataTypeStr=boolean
  Compare To Constant2 : simulink/Logic and Bit Operations/Compare To Constant  relop=<=  const=set_time2  OutDataTypeStr=boolean
  Compare To Constant3 : simulink/Logic and Bit Operations/Compare To Constant  relop=<=  const=set_time3  OutDataTypeStr=boolean
  D : Constant  Value=position_D
  Data Type Conversion : DataTypeConversion  OutDataTypeStr=uint32  SaturateOnIntegerOverflow=off  RndMeth=Floor
  Enabled Subsystem (PID setting) : Subsystem  TreatAsAtomicUnit=on
  Enabled Subsystem (initialization angle) : Subsystem  TreatAsAtomicUnit=on
  Enabled Subsystem (max current setting) : Subsystem  TreatAsAtomicUnit=on
  Enabled Subsystem (mode setting) : Subsystem  TreatAsAtomicUnit=on
  I : Constant  Value=position_I
  I2C Write (0x80) : arduinolib/I2C Write  I2CModule=0  Mode=Master  SlaveAddress=I2CAddress  SlaveByteOrder=LittleEndian  Direction=Transmitter  RegisterAddressMode=on  RegisterAddress=0x80  SlaveDataType=uint8  DataLength=1  NoAck=off  RepeatedStart=off  OutputStatus=off  blockPlatform=ARDUINO
  P : Constant  Value=position_P
  Sum : Sum  Inputs=++|
  max_current : Constant  Value=max_current
  position mode : Constant  Value=2
  rad to deg : Gain  Gain=180/pi
  x 100 : Gain  Gain=100
  wires:
  Enabled Subsystem (initialization angle)/1(initial angle) -> Sum/1
  command [rad]/1 -> rad to deg/1
  x 100/1 -> Data Type Conversion/1
  Sum/1 -> x 100/1
  Data Type Conversion/1 -> I2C Write (0x80)/1
  rad to deg/1 -> Sum/2
  Clock2/1 -> Compare To Constant2/1
  D/1 -> Enabled Subsystem (PID setting)/3(D)
  Compare To Constant1/1 -> Enabled Subsystem (mode setting)/Enable
  I/1 -> Enabled Subsystem (PID setting)/2(I)
  Clock1/1 -> Compare To Constant1/1
  position mode/1 -> Enabled Subsystem (mode setting)/1(mode)
  Compare To Constant3/1 -> Enabled Subsystem (max current setting)/Enable
  Clock3/1 -> Compare To Constant3/1
  P/1 -> Enabled Subsystem (PID setting)/1(P)
  max_current/1 -> Enabled Subsystem (max current setting)/1(max_current)
  Compare To Constant2/1 -> Enabled Subsystem (PID setting)/Enable
  Compare To Constant1-2/1 -> Enabled Subsystem (initialization angle)/Enable
  Clock1-2/1 -> Compare To Constant1-2/1
